simulink subsystem "LevMag_lineal"  (R2021a)
settings: Solver=VariableStepAuto  StartTime=0.0  StopTime=10.0  RelTol=1e-3
settings Model: Creator=zeta  LastModifiedBy=zeta

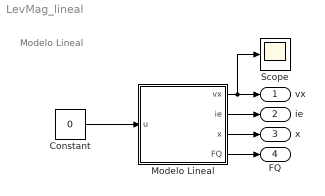
== system LevMag_lineal ==
  note: Modelo Lineal
  Constant : Constant  Value=0
  Modelo Lineal : Subsystem  mask{Ka=3, Km=1, K1=5888, K2=1536, R=20, L=0.2, uQ=0, xQ=3.2, vxQ=0, ieQ=0, vx_sat_sup=0, vx_sat_inf=-10, x_sat_sup=10, x_sat_inf=0, m=0.15, g=0}
      mask prompts: g "1000"
      mask DialogControl Control2 Prompt: Punto de operación:
      mask DialogControl Control3 Prompt: Saturación:
      mask DialogControl Control4 Prompt: otros
  Scope : Scope
  vx : Outport
  ie : Outport  Port=2
  x : Outport  Port=3
  FQ : Outport  Port=4
  wires:
  Constant/1 -> Modelo Lineal/1(u)
  Modelo Lineal/2(ie) -> ie/1
  Modelo Lineal/3(x) -> x/1
  Modelo Lineal/4(FQ) -> FQ/1
  Modelo Lineal/1(vx) -> Scope/1, vx/1

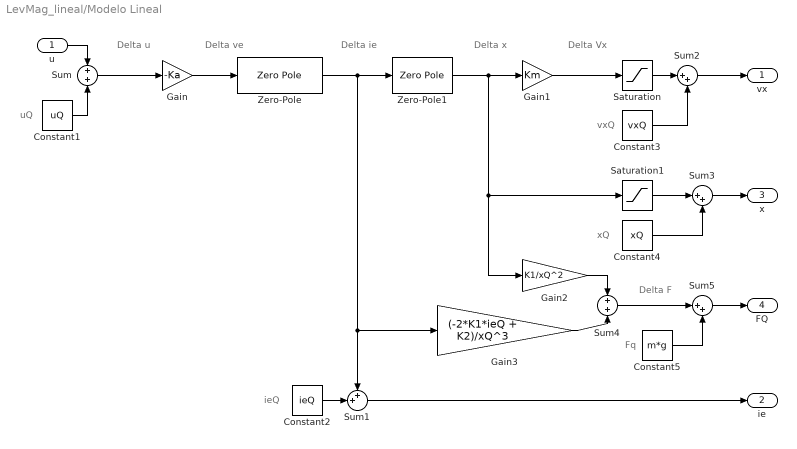
== system LevMag_lineal/Modelo Lineal ==
  note: Fq
  note: Delta F
  note: vxQ
  note: Delta Vx
  note: Delta x
  note: Delta ie
  note: Delta ve
  note: Delta u
  note: uQ
  note: ieQ
  note: xQ
  u : Inport
  Constant1 : Constant  Value=uQ
  Constant2 : Constant  Value=ieQ
  Constant3 : Constant  Value=vxQ
  Constant4 : Constant  Value=xQ
  Constant5 : Constant  Value=m*g
  Gain : Gain  Gain=-Ka
  Gain1 : Gain  Gain=Km
  Gain2 : Gain  Gain=K1/xQ^2
  Gain3 : Gain  Gain=(-2*K1*ieQ + K2)/xQ^3
  Saturation : Saturate  UpperLimit=vx_sat_sup  LowerLimit=vx_sat_inf
  Saturation1 : Saturate  UpperLimit=x_sat_sup  LowerLimit=x_sat_inf
  Sum : Sum  Inputs=+|+
  Sum1 : Sum  Inputs=++|
  Sum2 : Sum  Inputs=|++
  Sum3 : Sum  Inputs=|++
  Sum4 : Sum  Inputs=+|+
  Sum5 : Sum  Inputs=|++
  Zero-Pole : ZeroPole  Poles=[1 R/L]  Gain=[1/L]
  Zero-Pole1 : ZeroPole  Poles=[1 0 2*(K1*ieQ + K2)/m*xQ^3 ]  Gain=[-K1/ (m*xQ^2) ]
  vx : Outport
  ie : Outport  Port=2
  x : Outport  Port=3
  FQ : Outport  Port=4
  wires:
  u/1 -> Sum/1
  Sum1/1 -> ie/1
  Sum3/1 -> x/1
  Constant2/1 -> Sum1/2
  Constant4/1 -> Sum3/2
  Sum2/1 -> vx/1
  Sum4/1 -> Sum5/1
  Gain1/1 -> Saturation/1
  Saturation/1 -> Sum2/1
  Zero-Pole1/1 -> Gain1/1, Saturation1/1, Gain2/1
  Gain2/1 -> Sum4/1
  Constant5/1 -> Sum5/2
  Gain3/1 -> Sum4/2
  Zero-Pole/1 -> Sum1/1, Gain3/1, Zero-Pole1/1
  Saturation1/1 -> Sum3/1
  Sum5/1 -> FQ/1
  Constant1/1 -> Sum/2
  Sum/1 -> Gain/1
  Gain/1 -> Zero-Pole/1
  Constant3/1 -> Sum2/2
